simulink model "Team_Aura"  (R2024b)
settings: Solver=VariableStepAuto  StartTime=0.0  StopTime=10.0  RelTol=1e-3
libraries: spsThreePhaseVIMeasurementLib x6, spsThreePhaseTransformerTwoWindingsLib x5, spsThreePhaseBreakerLib x5, spsThreePhaseSourceLib x3, dspstat3 x2, spsThreePhaseParallelRLCBranchLib x1, sps_lib x1
settings Model: Creator=User  LastModifiedBy=User

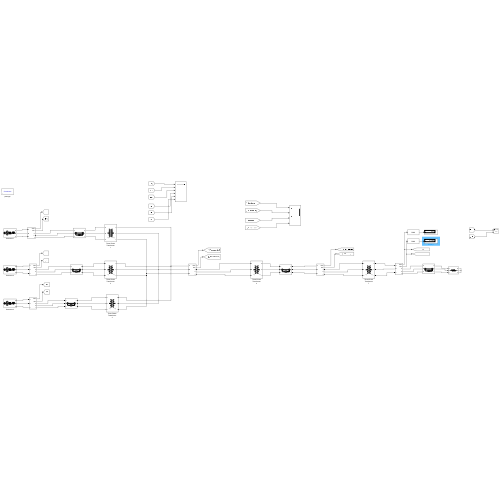
[thumbnail: Simulink's stored preview of the top-level diagram]
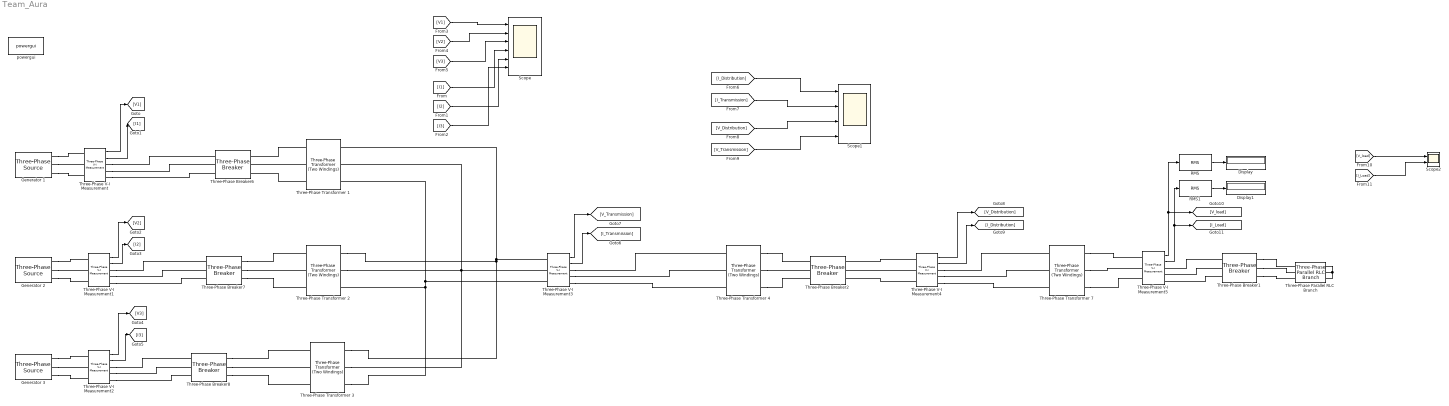
== system Team_Aura ==
  Display : Display
  Display1 : Display
  Generator 1 : spsThreePhaseSourceLib/Three-Phase Source  InternalConnection=Yg  VoltagePhases=off  Voltage=11e3  PhaseAngle=0  Voltage_phases=[25e3 25e3 25e3]/sqrt(3)  PhaseAngles_phases=[0 -120 +120]  Frequency=50  NonIdealSource=on  SpecifyImpedance=off  Resistance=0.8  Inductance=16.58e-3  ShortCircuitLevel=100e6  BaseVoltage=11e3  XRratio=7  BusType=PV  Pref=1000e3  Qref=0  Prefabc=[10e3, 10e3, 10e3]  Qrefabc=[0, 0, 0]  Qmin=-inf  Qmax=inf
  Generator 2 : spsThreePhaseSourceLib/Three-Phase Source  InternalConnection=Yg  VoltagePhases=off  Voltage=12e3  PhaseAngle=0  Voltage_phases=[25e3 25e3 25e3]/sqrt(3)  PhaseAngles_phases=[0 -120 +120]  Frequency=50  NonIdealSource=on  SpecifyImpedance=off  Resistance=0.8  Inductance=16.58e-3  ShortCircuitLevel=100e6  BaseVoltage=12e3  XRratio=7  BusType=PV  Pref=2000e3  Qref=0  Prefabc=[10e3, 10e3, 10e3]  Qrefabc=[0, 0, 0]  Qmin=-inf  Qmax=inf
  Generator 3 : spsThreePhaseSourceLib/Three-Phase Source  InternalConnection=Yg  VoltagePhases=off  Voltage=10e3  PhaseAngle=0  Voltage_phases=[25e3 25e3 25e3]/sqrt(3)  PhaseAngles_phases=[0 -120 +120]  Frequency=50  NonIdealSource=on  SpecifyImpedance=off  Resistance=0.8  Inductance=16.58e-3  ShortCircuitLevel=100e6  BaseVoltage=10e3  XRratio=7  BusType=PV  Pref=4000e3  Qref=0  Prefabc=[10e3, 10e3, 10e3]  Qrefabc=[0, 0, 0]  Qmin=-inf  Qmax=inf
  RMS : dspstat3/RMS  run=off  directionMode=Each column  dimension=1  InputProcessing=Columns as channels (frame based)  reset_popup=None
  RMS1 : dspstat3/RMS  run=off  directionMode=Each column  dimension=1  InputProcessing=Columns as channels (frame based)  reset_popup=None
  Scope : Scope  NumInputPorts=6
  Scope1 : Scope  NumInputPorts=4
  Scope2 : Scope  NumInputPorts=2
  Three-Phase Parallel RLC Branch : spsThreePhaseParallelRLCBranchLib/Three-Phase Parallel RLC Branch  LConnTagsString=A|B|C  RConnTagsString=A|B|C  BranchType=R  Resistance=5000  Inductance=1e-3  Capacitance=1e-6  Measurements=None
  Three-Phase Transformer 1 : spsThreePhaseTransformerTwoWindingsLib/Three-Phase Transformer (Two Windings)  Winding1Connection=Yg  Winding2Connection=Yg  CoreType=Three single-phase transformers  SetSaturation=off  Hysteresis=off  DataFile='hysteresis'  SetInitialFlux=off  Measurements=None  UNITS=pu  NominalPower=[ 2e6 , 50 ]  Winding1=[ 11e3 , 0.002 , 0.08 ]  Winding2=[ 132e3 , 0.002 , 0.08 ]  Rm=500  Lm=500  L0=0.5  Saturation=[ 0,0 ; 0.0024,1.2 ; 1.0,1.52 ]  InitialFluxes=[ 0.8 , -0.8 , 0.7 ]  BreakLoop=off  DiscreteSolver=Trapezoidal iterative  DataType=off  TransfoNumber=1
  Three-Phase Transformer 2 : spsThreePhaseTransformerTwoWindingsLib/Three-Phase Transformer (Two Windings)  Winding1Connection=Yg  Winding2Connection=Yg  CoreType=Three single-phase transformers  SetSaturation=off  Hysteresis=off  DataFile='hysteresis'  SetInitialFlux=off  Measurements=None  UNITS=pu  NominalPower=[ 3e6 , 50 ]  Winding1=[ 12e3 , 0.002 , 0.08 ]  Winding2=[ 132e3 , 0.002 , 0.08 ]  Rm=500  Lm=500  L0=0.5  Saturation=[ 0,0 ; 0.0024,1.2 ; 1.0,1.52 ]  InitialFluxes=[ 0.8 , -0.8 , 0.7 ]  BreakLoop=off  DiscreteSolver=Trapezoidal iterative  DataType=off  TransfoNumber=1
  Three-Phase Transformer 3 : spsThreePhaseTransformerTwoWindingsLib/Three-Phase Transformer (Two Windings)  Winding1Connection=Yg  Winding2Connection=Yg  CoreType=Three single-phase transformers  SetSaturation=off  Hysteresis=off  DataFile='hysteresis'  SetInitialFlux=off  Measurements=None  UNITS=pu  NominalPower=[ 5e6 , 50 ]  Winding1=[ 10e3 , 0.002 , 0.08 ]  Winding2=[ 132e3 , 0.002 , 0.08 ]  Rm=500  Lm=500  L0=0.5  Saturation=[ 0,0 ; 0.0024,1.2 ; 1.0,1.52 ]  InitialFluxes=[ 0.8 , -0.8 , 0.7 ]  BreakLoop=off  DiscreteSolver=Trapezoidal iterative  DataType=off  TransfoNumber=1
  Three-Phase Transformer 4 : spsThreePhaseTransformerTwoWindingsLib/Three-Phase Transformer (Two Windings)  Winding1Connection=Yg  Winding2Connection=Yg  CoreType=Three single-phase transformers  SetSaturation=off  Hysteresis=off  DataFile='hysteresis'  SetInitialFlux=off  Measurements=None  UNITS=pu  NominalPower=[ 10e6 , 50 ]  Winding1=[ 132e3 , 0.002 , 0.08 ]  Winding2=[ 11e3 , 0.002 , 0.08 ]  Rm=500  Lm=500  L0=0.5  Saturation=[ 0,0 ; 0.0024,1.2 ; 1.0,1.52 ]  InitialFluxes=[ 0.8 , -0.8 , 0.7 ]  BreakLoop=off  DiscreteSolver=Trapezoidal iterative  DataType=off  TransfoNumber=1
  Three-Phase Transformer 7 : spsThreePhaseTransformerTwoWindingsLib/Three-Phase Transformer (Two Windings)  Winding1Connection=Yg  Winding2Connection=Yg  CoreType=Three single-phase transformers  SetSaturation=off  Hysteresis=off  DataFile='hysteresis'  SetInitialFlux=off  Measurements=None  UNITS=pu  NominalPower=[ 10e6 , 50 ]  Winding1=[ 11e3 , 0.002 , 0.08 ]  Winding2=[ 400 , 0.002 , 0.08 ]  Rm=500  Lm=500  L0=0.5  Saturation=[ 0,0 ; 0.0024,1.2 ; 1.0,1.52 ]  InitialFluxes=[ 0.8 , -0.8 , 0.7 ]  BreakLoop=off  DiscreteSolver=Trapezoidal iterative  DataType=off  TransfoNumber=1
  Three-Phase V-I Measurement{,1..5} (6 alike) : spsThreePhaseVIMeasurementLib/Three-Phase V-I Measurement  VoltageMeasurement=phase-to-ground  SetLabelV=off  LabelV=Vabc  Vpu=off  VpuLL=off  CurrentMeasurement=yes  SetLabelI=off  LabelI=Iabc  Ipu=off  Pbase=100e6  Vbase=500e3  OutputType=Complex  PhasorSimulation=off  PSBequivalent=0
  Three-Phase Breaker{1..2,6..8} (5 alike) : spsThreePhaseBreakerLib/Three-Phase Breaker  InitialState=closed  SwitchA=on  SwitchB=on  SwitchC=on  SwitchTimes="[1/60  5/60]"  External=off  BreakerResistance=0.01  SnubberResistance=1e6  SnubberCapacitance=inf  Measurements=None
  powergui : sps_lib/powergui  Priority=1  SimulationMode=Continuous  SampleTime=50e-6  frequency=60  Iterations=50  frequencyindice=50  Pbase=100e6  ErrMax=1e-4  UnitsV=kV  UnitsW=MW  buscounter=0  FunctionMessages=off  echomessages=off  EnableUseOfTLC=off  CurrentSourceSwitches=off  DisableSnubberDevices=off  DisableRonSwitches=off  DisableVfSwitches=off  DisplayEquations=off  AutomaticDiscreteSolvers=off  SolverType=Tustin/Backward Euler (TBE)  Interpol=off  ExternalGateDelay=off  methode=off  Ts=100  x0status=blocks  SPID=on  SwTol=0  HookPort=off  NonlinearTolerance=1e-4  nMaxIteration=100  ContinueOnMaxIteration=off  RestoreLinks=warning  ResistiveCurrentMeasurement=off  Frange=[0:2:500]  Ylog=off  Xlog=on  ShowGrid=off  save=off  variable=ZData  structure=0  ZoomFFT=off  StartTime=0.0  cycles=1  DisplayStyle=1  fundamental=60  FreqAxis=off  MaxFrequency=1000  frequencyindicesteady=1  RmsSteady=1  display=off
  wires:
  Three-Phase V-I Measurement/1 -> [V1]
  Three-Phase V-I Measurement/2 -> [I1]
  Three-Phase V-I Measurement1/1 -> [V2]
  Three-Phase V-I Measurement1/2 -> [I2]
  Three-Phase V-I Measurement2/2 -> [I3]
  Three-Phase V-I Measurement2/1 -> [V3]
  Three-Phase V-I Measurement3/2 -> [I_Transmission]
  Three-Phase V-I Measurement3/1 -> [V_Transmission]
  Three-Phase V-I Measurement4/2 -> [I_Distribution]
  Three-Phase V-I Measurement4/1 -> [V_Distribution]
  [V1] -> Scope/1
  [V2] -> Scope/2
  [V3] -> Scope/3
  [I1] -> Scope/4
  [I2] -> Scope/5
  [I3] -> Scope/6
  [I_Transmission] -> Scope1/2
  [V_Distribution] -> Scope1/3
  [I_Distribution] -> Scope1/1
  [V_Transmission] -> Scope1/4
  Three-Phase V-I Measurement5/2 -> RMS1/1, [I_Load]
  Three-Phase V-I Measurement5/1 -> RMS/1, [V_load]
  [V_load] -> Scope2/1
  [I_Load] -> Scope2/2
  RMS/1 -> Display/1
  RMS1/1 -> Display1/1
  connections:
  Three-Phase Transformer 4/RConn1 -- Three-Phase Breaker2/LConn1
  Three-Phase Transformer 4/RConn3 -- Three-Phase Breaker2/LConn3
  Three-Phase Transformer 4/RConn2 -- Three-Phase Breaker2/LConn2
  Three-Phase Transformer 2/RConn2 -- Three-Phase Transformer 1/RConn2 -- Three-Phase V-I Measurement3/LConn2 -- Three-Phase Transformer 3/RConn2
  Three-Phase Transformer 1/RConn1 -- Three-Phase Transformer 3/RConn1 -- Three-Phase Transformer 2/RConn1 -- Three-Phase V-I Measurement3/LConn1
  Three-Phase Transformer 1/RConn3 -- Three-Phase V-I Measurement3/LConn3 -- Three-Phase Transformer 3/RConn3 -- Three-Phase Transformer 2/RConn3
  Three-Phase V-I Measurement4/LConn2 -- Three-Phase Breaker2/RConn2
  Three-Phase V-I Measurement4/LConn1 -- Three-Phase Breaker2/RConn1
  Three-Phase V-I Measurement4/LConn3 -- Three-Phase Breaker2/RConn3
  Three-Phase V-I Measurement4/RConn3 -- Three-Phase Transformer 7/LConn3
  Three-Phase V-I Measurement4/RConn2 -- Three-Phase Transformer 7/LConn2
  Three-Phase V-I Measurement4/RConn1 -- Three-Phase Transformer 7/LConn1
  Three-Phase Parallel RLC Branch/RConn1 -- Three-Phase Parallel RLC Branch/RConn2 -- Three-Phase Parallel RLC Branch/RConn3
  Generator 1/RConn2 -- Three-Phase V-I Measurement/LConn2
  Generator 1/RConn1 -- Three-Phase V-I Measurement/LConn1
  Generator 1/RConn3 -- Three-Phase V-I Measurement/LConn3
  Three-Phase V-I Measurement/RConn3 -- Three-Phase Breaker6/LConn3
  Three-Phase V-I Measurement/RConn2 -- Three-Phase Breaker6/LConn2
  Three-Phase V-I Measurement/RConn1 -- Three-Phase Breaker6/LConn1
  Three-Phase Transformer 1/LConn2 -- Three-Phase Breaker6/RConn2
  Three-Phase Transformer 1/LConn1 -- Three-Phase Breaker6/RConn1
  Three-Phase Transformer 1/LConn3 -- Three-Phase Breaker6/RConn3
  Generator 2/RConn2 -- Three-Phase V-I Measurement1/LConn2
  Generator 2/RConn1 -- Three-Phase V-I Measurement1/LConn1
  Generator 2/RConn3 -- Three-Phase V-I Measurement1/LConn3
  Three-Phase V-I Measurement1/RConn3 -- Three-Phase Breaker7/LConn3
  Three-Phase V-I Measurement1/RConn2 -- Three-Phase Breaker7/LConn2
  Three-Phase V-I Measurement1/RConn1 -- Three-Phase Breaker7/LConn1
  Three-Phase Breaker7/RConn2 -- Three-Phase Transformer 2/LConn2
  Three-Phase Breaker7/RConn1 -- Three-Phase Transformer 2/LConn1
  Three-Phase Breaker7/RConn3 -- Three-Phase Transformer 2/LConn3
  Generator 3/RConn2 -- Three-Phase V-I Measurement2/LConn2
  Generator 3/RConn1 -- Three-Phase V-I Measurement2/LConn1
  Generator 3/RConn3 -- Three-Phase V-I Measurement2/LConn3
  Three-Phase V-I Measurement2/RConn3 -- Three-Phase Breaker8/LConn3
  Three-Phase V-I Measurement2/RConn2 -- Three-Phase Breaker8/LConn2
  Three-Phase V-I Measurement2/RConn1 -- Three-Phase Breaker8/LConn1
  Three-Phase Breaker8/RConn2 -- Three-Phase Transformer 3/LConn2
  Three-Phase Breaker8/RConn1 -- Three-Phase Transformer 3/LConn1
  Three-Phase Breaker8/RConn3 -- Three-Phase Transformer 3/LConn3
  Three-Phase V-I Measurement3/RConn3 -- Three-Phase Transformer 4/LConn3
  Three-Phase V-I Measurement3/RConn2 -- Three-Phase Transformer 4/LConn2
  Three-Phase V-I Measurement3/RConn1 -- Three-Phase Transformer 4/LConn1
  Three-Phase Transformer 7/RConn2 -- Three-Phase V-I Measurement5/LConn2
  Three-Phase Transformer 7/RConn1 -- Three-Phase V-I Measurement5/LConn1
  Three-Phase Transformer 7/RConn3 -- Three-Phase V-I Measurement5/LConn3
  Three-Phase Breaker1/LConn3 -- Three-Phase V-I Measurement5/RConn3
  Three-Phase Breaker1/LConn2 -- Three-Phase V-I Measurement5/RConn2
  Three-Phase Breaker1/LConn1 -- Three-Phase V-I Measurement5/RConn1
  Three-Phase Breaker1/RConn1 -- Three-Phase Parallel RLC Branch/LConn1
  Three-Phase Breaker1/RConn2 -- Three-Phase Parallel RLC Branch/LConn2
  Three-Phase Breaker1/RConn3 -- Three-Phase Parallel RLC Branch/LConn3
